simulink model "commandGeneration_test"  (R2018b)
settings: Solver=VariableStepAuto  StartTime=0.0  StopTime=600  RelTol=1e-3
undefined symbols (not defined in the file): simParams
libraries: rpm_2_torque_lib x4, pd_processing_lib x1, solar_panels_lib x1, sun_sensor_lib x1, MEKF_Conversion_lib x1, controlSelection_lib x1, quat_err_lib x1, quat_kinematics_lib x1, rigid_body_dynamics_lib x1
settings Model: Creator=colem  LastModifiedBy=Taylor

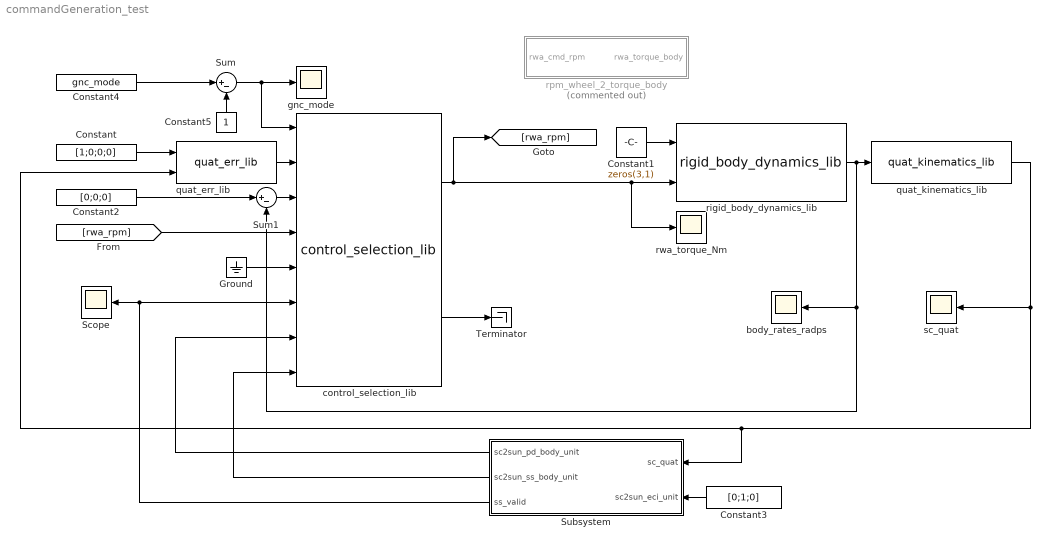
== system commandGeneration_test ==
  Constant : Constant  Value=[1;0;0;0]
  Constant1 : Constant  Value=zeros(3,1)
  Constant2 : Constant  Value=[0;0;0]
  Constant3 : Constant  Value=[0;1;0]
  Constant4 : Constant  Value=gnc_mode  mask{gnc_mode=5}
      mask prompts: gnc_mode "GNC mode"
      mask TypeOptions gnc_mode: 0 | 1 | 2 | 3 | 4 | 5 | 6 | 7 | 8
      mask DialogControl DescTextVar Prompt: Set the GNC mode to verify performance of various controllers.
  Constant5 : Constant
  Ground : Ground
  Scope : Scope
  Subsystem : Subsystem
  Sum : Sum  Inputs=|+-
  Sum1 : Sum  Inputs=|+-
  Terminator : Terminator
  body_rates_radps : Scope
  control_selection_lib : controlSelection_lib/control_selection_lib  SystemSampleTime=-1
  gnc_mode : Scope
  quat_err_lib : quat_err_lib/quat_err_lib  SystemSampleTime=-1
  quat_kinematics_lib : quat_kinematics_lib/quat_kinematics_lib  SystemSampleTime=-1
  rigid_body_dynamics_lib : rigid_body_dynamics_lib/rigid_body_dynamics_lib  SystemSampleTime=-1
  rpm_wheel_2_torque_body : Subsystem  Commented=on
  rwa_torque_Nm : Scope
  sc_quat : Scope
  wires:
  Constant/1 -> quat_err_lib/1
  rigid_body_dynamics_lib/1 -> Sum1/2, body_rates_radps/1, quat_kinematics_lib/1
  control_selection_lib/2 -> Terminator/1
  Constant1/1 -> rigid_body_dynamics_lib/1
  Ground/1 -> control_selection_lib/5
  [rwa_rpm] -> control_selection_lib/4
  Constant2/1 -> Sum1/1
  quat_kinematics_lib/1 -> Subsystem/1(sc_quat), quat_err_lib/2, sc_quat/1
  control_selection_lib/1 -> rwa_torque_Nm/1, rigid_body_dynamics_lib/2, [rwa_rpm]
  Constant4/1 -> Sum/1
  Sum/1 -> control_selection_lib/1, gnc_mode/1
  Constant5/1 -> Sum/2
  quat_err_lib/1 -> control_selection_lib/2
  Sum1/1 -> control_selection_lib/3
  Constant3/1 -> Subsystem/2(sc2sun_eci_unit)
  Subsystem/3(ss_valid) -> control_selection_lib/6, Scope/1
  Subsystem/2(sc2sun_ss_body_unit) -> control_selection_lib/8
  Subsystem/1(sc2sun_pd_body_unit) -> control_selection_lib/7

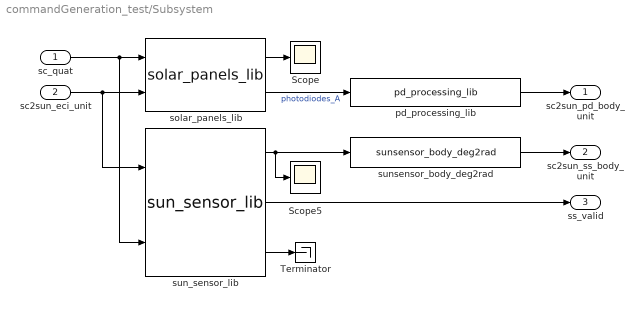
== system commandGeneration_test/Subsystem ==
  sc_quat : Inport
  sc2sun_eci_unit : Inport  Port=2
  Scope : Scope
  Scope5 : Scope
  Terminator : Terminator
  pd_processing_lib : pd_processing_lib/pd_processing_lib  SystemSampleTime=-1
  solar_panels_lib : solar_panels_lib/solar_panels_lib  SystemSampleTime=-1
  "sun_sensor_lib " : sun_sensor_lib/sun_sensor_lib   SystemSampleTime=-1
  sunsensor_body_deg2rad : MEKF_Conversion_lib/Conversion_lib/sunsensor_body_deg2rad  SystemSampleTime=-1
  sc2sun_pd_body_unit : Outport
  sc2sun_ss_body_unit : Outport  Port=2
  ss_valid : Outport  Port=3
  wires:
  "sun_sensor_lib "/2 -> ss_valid/1
  pd_processing_lib/1 -> sc2sun_pd_body_unit/1
  sunsensor_body_deg2rad/1 -> sc2sun_ss_body_unit/1
  solar_panels_lib/1 -> Scope/1
  "sun_sensor_lib "/3 -> Terminator/1
  "sun_sensor_lib "/1 -> sunsensor_body_deg2rad/1, Scope5/1
  sc_quat/1 -> solar_panels_lib/1, "sun_sensor_lib "/2
  solar_panels_lib/2 -> pd_processing_lib/1  "photodiodes_A"
  sc2sun_eci_unit/1 -> "sun_sensor_lib "/1, solar_panels_lib/2

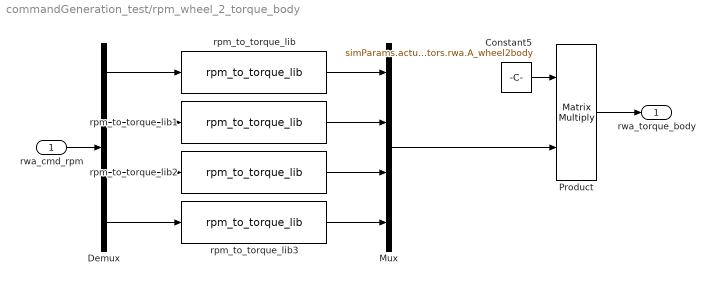
== system commandGeneration_test/rpm_wheel_2_torque_body ==
  rwa_cmd_rpm : Inport
  Constant5 : Constant  Value=simParams.actuators.rwa.A_wheel2body
  Demux : Demux
  Mux : Mux
  Product : Product  Multiplication=Matrix(*)
  rpm_to_torque_lib{,1..3} (4 alike) : rpm_2_torque_lib/rpm_to_torque_lib  SystemSampleTime=-1
  rwa_torque_body : Outport
  wires:
  rwa_cmd_rpm/1 -> Demux/1
  Demux/1 -> rpm_to_torque_lib/1
  Demux/2 -> rpm_to_torque_lib1/1
  Demux/3 -> rpm_to_torque_lib2/1
  Demux/4 -> rpm_to_torque_lib3/1
  rpm_to_torque_lib3/1 -> Mux/4
  rpm_to_torque_lib1/1 -> Mux/2
  rpm_to_torque_lib/1 -> Mux/1
  rpm_to_torque_lib2/1 -> Mux/3
  Mux/1 -> Product/2
  Constant5/1 -> Product/1
  Product/1 -> rwa_torque_body/1
